simulink model "PID_digital_tarea"  (R2021a)
settings: Solver=ode45  StartTime=0.0  StopTime=10  MaxStep=1e-5  RelTol=1e-3  EnableMultiTasking=on
values from neighbouring files (symbols this model uses):
  P = [-2 0]    [Tp2_Laboret.m]
  Tm = 0.06    [Tp2_Laboret.m]
undefined symbols (not defined in the file or in its folder): DiscIntNeverNeededParam
libraries: simulink x1
settings Model: Creator=Usuario  LastModifiedBy=Guada
settings SolverCC: AlgebraicLoopSolver=TrustRegion
settings DataIOCC: SaveFormat=Array  SignalLoggingSaveFormat=ModelDataLogs  ReturnWorkspaceOutputs=off
settings OptimizationCC: InitFltsAndDblsToZero=on  LifeSpan=inf
settings DebuggingCC: SaveWithParameterizedLinksMsg=none  UnderspecifiedInitializationDetection=Classic  MergeDetectMultiDrivingBlocksExec=none  SignalResolutionControl=TryResolveAllWithWarning  SolverPrmCheckMsg=warning  MultiTaskDSMMsg=warning  MultiTaskCondExecSysMsg=none  FcnCallInpInsideContextMsg=warning  SFUnexpectedBacktrackingDiag=warning  SFNoUnconditionalDefaultTransitionDiag=warning  SFExecutionAtInitializationDiag=none  SFMachineParentedDataDiag=warning  ArithmeticOperatorsInVariantConditions=warning
settings HardwareCC: ProdBitPerPointer=32  ProdBitPerSizeT=32  ProdBitPerPtrDiffT=32  ProdLargestAtomicFloat=None  ProdIntDivRoundTo=Undefined  ProdEndianess=Unspecified  ProdWordSize=32  ProdHWDeviceType=32-bit Generic
settings ModelReferenceCC: PropagateSignalLabelsOutOfModel=off
settings SFSimCC: SimUseLocalCustomCode=off  CustomCodeUndefinedFunction=UseInterfaceOnly
settings RTWCC: RTWUseLocalCustomCode=off
settings CodeAppCC: StateflowObjectComments=on
settings GRTTargetCC: TargetFcnLib=ansi_tfl_tmw.mat  TargetLangStandard=C89/C90 (ANSI)  CombineOutputUpdateFcns=off  GRTInterface=on
settings ConfigComp: CovMetricSettings=dw  CovSaveCumulativeToWorkspaceVar=on  CovSaveSingleToWorkspaceVar=on  CovExternalEMLEnable=off  CovSFcnEnable=off

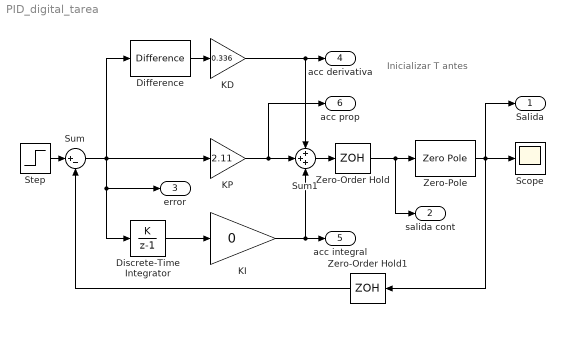
== system PID_digital_tarea ==
  note: Inicializar T antes
  Difference : simulink/Discrete/Difference  ICPrevInput=0.0  OutMin=[]  OutMax=[]  OutDataType=fixdt(1, 16)  OutScaling=2^-10  DoSatur=off
  Discrete-Time Integrator : DiscreteIntegrator  IntegratorMethod=Accumulation: Forward Euler  SampleTime=-1  ICPrevOutput=DiscIntNeverNeededParam  ICPrevScaledInput=DiscIntNeverNeededParam
  KD : Gain  Gain=0.336
  KI : Gain  Gain=0
  KP : Gain  Gain=2.11
  Scope : Scope
  Step : Step  Time=Tm  SampleTime=Tm
  Sum : Sum  Inputs=|+-
  Sum1 : Sum  Inputs=+++
  Zero-Order Hold : ZeroOrderHold  SampleTime=Tm
  Zero-Order Hold1 : ZeroOrderHold  SampleTime=Tm
  Zero-Pole : ZeroPole  Zeros=[]  Poles=[P]  Gain=[5]
  Salida : Outport
  salida cont : Outport  Port=2
  error : Outport  Port=3
  acc derivativa : Outport  Port=4
  acc integral : Outport  Port=5
  acc prop : Outport  Port=6
  wires:
  Zero-Order Hold/1 -> Zero-Pole/1, salida cont/1
  Step/1 -> Sum/1
  Zero-Pole/1 -> Zero-Order Hold1/1, Scope/1, Salida/1
  KI/1 -> Sum1/3, acc integral/1
  KP/1 -> acc prop/1, Sum1/2
  Zero-Order Hold1/1 -> Sum/2
  Sum/1 -> Difference/1, Discrete-Time Integrator/1, error/1, KP/1
  Sum1/1 -> Zero-Order Hold/1
  KD/1 -> Sum1/1, acc derivativa/1
  Difference/1 -> KD/1
  Discrete-Time Integrator/1 -> KI/1
